simulink model "dc_motor_"  (R2023b)
settings: Solver=VariableStepAuto  StartTime=0.0  StopTime=0.05  RelTol=1e-3
values from neighbouring files (symbols this model uses):
  b = Jm / 0.00376    (= 0.00264627659574)    [homeworktwo.m]
  Jm = 0.00000995    (= 9.95e-06)    [homeworktwo.m]
  Ke = 0.0683    [homeworktwo.m]
  Kt = 0.0683    [homeworktwo.m]
  La = 0.000658    [homeworktwo.m]
  Ra = 1.76    [homeworktwo.m]
  Tl_ = 0    [homeworktwo.m]
  Va = 48    [homeworktwo.m]
settings Model: Creator=junseo  LastModifiedBy=minjs
settings OptimizationCC: ReuseModelBlockBuffer=off

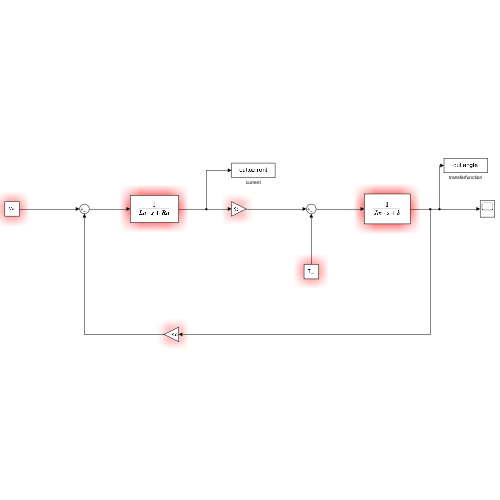
[thumbnail: Simulink's stored preview of the top-level diagram]
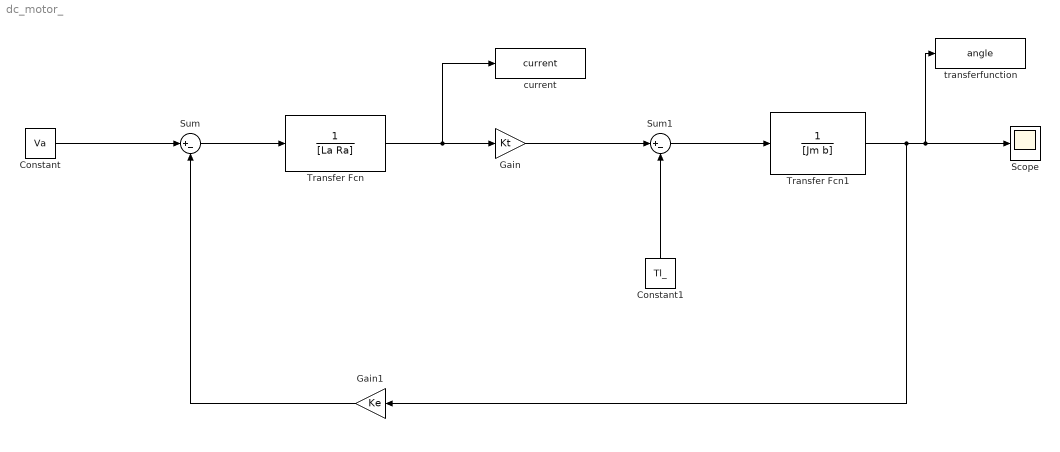
== system dc_motor_ ==
  Constant : Constant  Value=Va
  Constant1 : Constant  Value=Tl_
  Gain : Gain  Gain=Kt
  Gain1 : Gain  Gain=Ke
  Scope : Scope
  Sum : Sum  Inputs=|+-
  Sum1 : Sum  Inputs=|+-
  Transfer Fcn : TransferFcn  Denominator=[La Ra]
  Transfer Fcn1 : TransferFcn  Denominator=[Jm b]
  current : ToWorkspace  VariableName=current  SaveFormat=Timeseries  SampleTime=-1
  transferfunction : ToWorkspace  VariableName=angle  SaveFormat=Timeseries  SampleTime=-1
  wires:
  Constant/1 -> Sum/1
  Sum/1 -> Transfer Fcn/1
  Transfer Fcn/1 -> current/1, Gain/1
  Gain/1 -> Sum1/1
  Sum1/1 -> Transfer Fcn1/1
  Constant1/1 -> Sum1/2
  Transfer Fcn1/1 -> Gain1/1, transferfunction/1, Scope/1
  Gain1/1 -> Sum/2
